simulink model "Aircraft_Simulator_LAT"  (R2019b)
settings: Solver=ode4  StartTime=0.0  StopTime=tfinal  FixedStep=dt  RelTol=1e-3
undefined symbols (not defined in the file or in its folder): aircraft_data, F_gravity_0, initial_conditions, Ixx, Iyy, Izz, m, M0, Matrix_Controls, Matrix_states, s0
libraries: simulink_extras x8, shared6dof x1, aerolibasang x1
settings Model: Creator=yossef  LastModifiedBy=Yousef
settings DataIOCC: ReturnWorkspaceOutputs=off
settings DebuggingCC: ArithmeticOperatorsInVariantConditions=warning
settings SFSimCC: SimUseLocalCustomCode=off  CustomCodeUndefinedFunction=UseInterfaceOnly
settings RTWCC: RTWUseLocalCustomCode=off

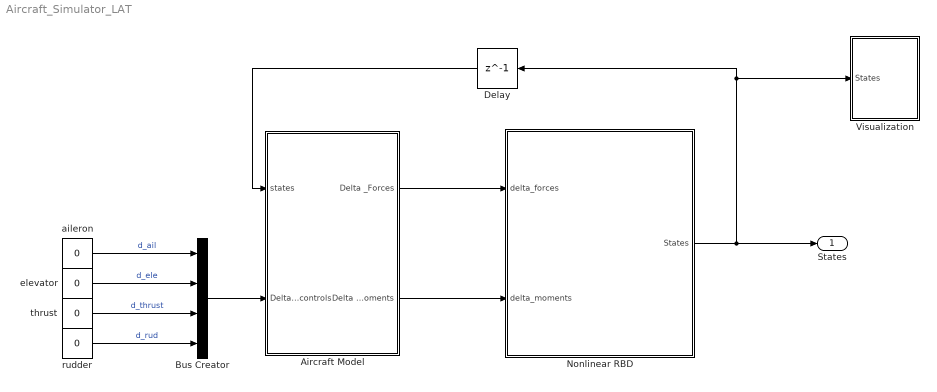
== system Aircraft_Simulator_LAT ==
  Aircraft Model : Subsystem
  Bus Creator : BusCreator  Inputs=4
  Delay : Delay  DelayLength=1  InitialCondition=initial_conditions
  Nonlinear RBD : Subsystem
  Visualization : Subsystem
  aileron : Constant  Value=0
  elevator : Constant  Value=0
  rudder : Constant  Value=0
  thrust : Constant  Value=0
  States : Outport
  wires:
  Delay/1 -> Aircraft Model/1(states)
  Nonlinear RBD/1(States) -> States/1, Delay/1, Visualization/1(States)
  Aircraft Model/1(Delta _Forces) -> Nonlinear RBD/1(delta_forces)
  Aircraft Model/2(Delta _Moments) -> Nonlinear RBD/2(delta_moments)
  aileron/1 -> Bus Creator/1  "d_ail"
  elevator/1 -> Bus Creator/2  "d_ele"
  thrust/1 -> Bus Creator/3  "d_thrust"
  rudder/1 -> Bus Creator/4  "d_rud"
  Bus Creator/1 -> Aircraft Model/2(Delta_controls)

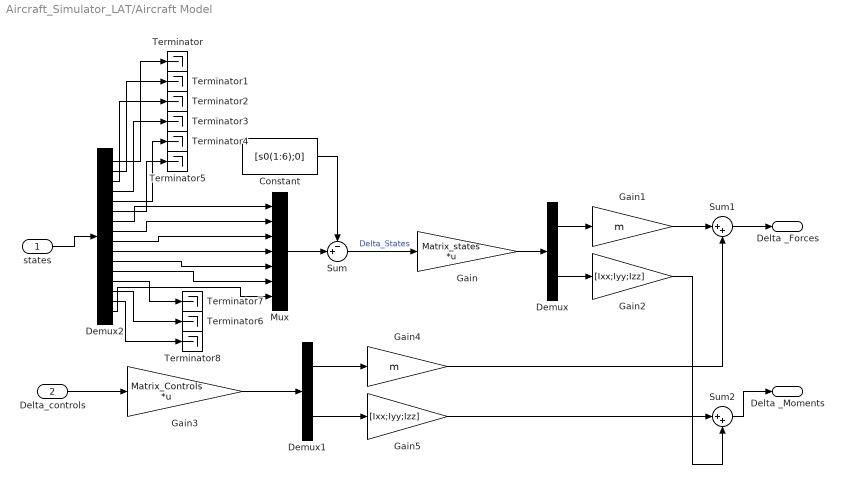
== system Aircraft_Simulator_LAT/Aircraft Model ==
  states : Inport
  Delta_controls : Inport  Port=2
  Constant : Constant  Value=[s0(1:6);0]
  Demux : Demux  Outputs=2
  Demux1 : Demux  Outputs=2
  Demux2 : Demux  Outputs=16
  Gain : Gain  Gain=Matrix_states  Multiplication=Matrix(K*u)
  Gain1 : Gain  Gain=m
  Gain2 : Gain  Gain=[Ixx;Iyy;Izz]
  Gain3 : Gain  Gain=Matrix_Controls  Multiplication=Matrix(K*u)
  Gain4 : Gain  Gain=m
  Gain5 : Gain  Gain=[Ixx;Iyy;Izz]
  Mux : Mux  Inputs=7
  Sum : Sum  Inputs=-+|
  Sum1 : Sum  Inputs=|++
  Sum2 : Sum  Inputs=|++
  Terminator{,1..8} (9 alike) : Terminator
  Delta _Forces : Outport
  Delta _Moments : Outport  Port=2
  wires:
  Mux/1 -> Sum/2
  Constant/1 -> Sum/1
  Sum/1 -> Gain/1  "Delta_States"
  Gain/1 -> Demux/1
  Demux/1 -> Gain1/1
  Demux/2 -> Gain2/1
  Gain2/1 -> Sum2/2
  Gain1/1 -> Sum1/1
  Sum1/1 -> Delta _Forces/1
  Sum2/1 -> Delta _Moments/1
  Delta_controls/1 -> Gain3/1
  Gain3/1 -> Demux1/1
  Demux1/1 -> Gain4/1
  Demux1/2 -> Gain5/1
  Gain4/1 -> Sum1/2
  Gain5/1 -> Sum2/1
  states/1 -> Demux2/1
  Demux2/1 -> Terminator/1
  Demux2/2 -> Terminator1/1
  Demux2/3 -> Terminator2/1
  Demux2/7 -> Mux/1
  Demux2/8 -> Mux/2
  Demux2/9 -> Mux/3
  Demux2/10 -> Mux/4
  Demux2/11 -> Mux/5
  Demux2/12 -> Mux/6
  Demux2/16 -> Mux/7
  Demux2/4 -> Terminator3/1
  Demux2/5 -> Terminator4/1
  Demux2/6 -> Terminator5/1
  Demux2/13 -> Terminator7/1
  Demux2/14 -> Terminator6/1
  Demux2/15 -> Terminator8/1

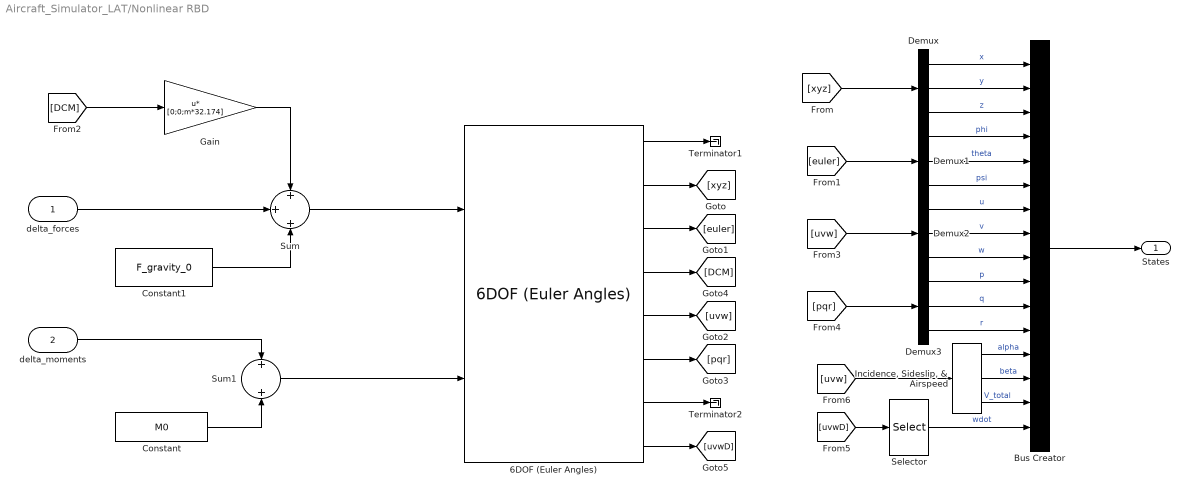
== system Aircraft_Simulator_LAT/Nonlinear RBD ==
  delta_forces : Inport
  delta_moments : Inport  Port=2
  6DOF (Euler Angles) : shared6dof/6DOF (Euler Angles)  units=English (Velocity in ft/s)  mtype=Fixed  rep=Euler Angles  xme_0=aircraft_data(13:15)  Vm_0=aircraft_data(4:6)  eul_0=aircraft_data(10:12)  pm_0=aircraft_data(7:9)  mass_0=m  mass_e=0.5  mass_f=2.0  inertia=I  inertia_e=eye(3)  inertia_f=2*eye(3)  k_quat=1.0  vre_flag=on  abi_flag=off  aMode=0  xme_statename=''  Vm_statename=''  eul_statename=''  quat_statename=''  pm_statename=''  mass_statename=''
      settings: SourceProductBaseCode=AE
  Bus Creator : BusCreator  Inputs=16
  Constant : Constant  Value=M0
  Constant1 : Constant  Value=F_gravity_0
  Demux{,1..3} (4 alike) : Demux  Outputs=3
  Gain : Gain  Gain=[0;0;m*32.174]  Multiplication=Matrix(u*K)
  "Incidence, Sideslip, & Airspeed" : aerolibasang/Incidence, Sideslip, & Airspeed
      settings: SourceProductName=Aerospace Blockset
  Selector : Selector  InputPortWidth=3  IndexOptions=Index vector (dialog)  Indices=[3]  OutputSizes=1
  Sum : Sum  Inputs=+||+||+
  Sum1 : Sum  Inputs=+||+
  Terminator1 : Terminator
  Terminator2 : Terminator
  States : Outport
  wires:
  6DOF (Euler Angles)/4 -> [DCM]
  6DOF (Euler Angles)/1 -> Terminator1/1
  6DOF (Euler Angles)/2 -> [xyz]
  6DOF (Euler Angles)/3 -> [euler]
  6DOF (Euler Angles)/5 -> [uvw]
  6DOF (Euler Angles)/6 -> [pqr]
  6DOF (Euler Angles)/7 -> Terminator2/1
  6DOF (Euler Angles)/8 -> [uvwD]
  Demux/2 -> Bus Creator/2  "y"
  [xyz] -> Demux/1
  Demux/1 -> Bus Creator/1  "x"
  Demux/3 -> Bus Creator/3  "z"
  [uvw] -> Demux2/1
  [pqr] -> Demux3/1
  Demux1/1 -> Bus Creator/4  "phi"
  Demux1/2 -> Bus Creator/5  "theta"
  Demux1/3 -> Bus Creator/6  "psi"
  Demux2/1 -> Bus Creator/7  "u"
  Demux2/2 -> Bus Creator/8  "v"
  Demux2/3 -> Bus Creator/9  "w"
  Demux3/1 -> Bus Creator/10  "p"
  Demux3/2 -> Bus Creator/11  "q"
  Demux3/3 -> Bus Creator/12  "r"
  "Incidence, Sideslip, & Airspeed"/1 -> Bus Creator/13  "alpha"
  "Incidence, Sideslip, & Airspeed"/2 -> Bus Creator/14  "beta"
  "Incidence, Sideslip, & Airspeed"/3 -> Bus Creator/15  "V_total"
  [uvw] -> "Incidence, Sideslip, & Airspeed"/1
  Selector/1 -> Bus Creator/16  "wdot"
  [uvwD] -> Selector/1
  Bus Creator/1 -> States/1
  Constant1/1 -> Sum/3
  [DCM] -> Gain/1
  Gain/1 -> Sum/1
  Sum/1 -> 6DOF (Euler Angles)/1
  delta_forces/1 -> Sum/2
  Constant/1 -> Sum1/2
  delta_moments/1 -> Sum1/1
  Sum1/1 -> 6DOF (Euler Angles)/2
  [euler] -> Demux1/1

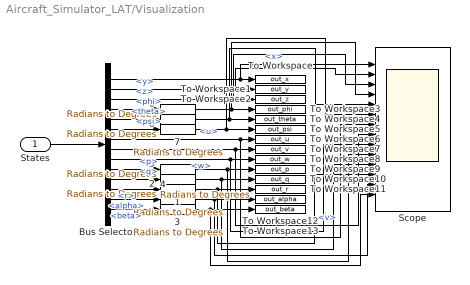
== system Aircraft_Simulator_LAT/Visualization ==
  States : Inport
  {1..8} (8 alike) : simulink_extras/Transformations/Radians to Degrees
  Bus Selector : BusSelector  OutputSignals=x,y,z,phi,theta,psi,u,v,w,p,q,r,alpha,beta
  Scope : Scope  NumInputPorts=14
  To Workspace : ToWorkspace  VariableName=out_x  SampleTime=-1
  To Workspace1 : ToWorkspace  VariableName=out_y  SampleTime=-1
  To Workspace10 : ToWorkspace  VariableName=out_q  SampleTime=-1
  To Workspace11 : ToWorkspace  VariableName=out_r  SampleTime=-1
  To Workspace12 : ToWorkspace  VariableName=out_alpha  SampleTime=-1
  To Workspace13 : ToWorkspace  VariableName=out_beta  SampleTime=-1
  To Workspace2 : ToWorkspace  VariableName=out_z  SampleTime=-1
  To Workspace3 : ToWorkspace  VariableName=out_phi  SampleTime=-1
  To Workspace4 : ToWorkspace  VariableName=out_theta  SampleTime=-1
  To Workspace5 : ToWorkspace  VariableName=out_psi  SampleTime=-1
  To Workspace6 : ToWorkspace  VariableName=out_u  SampleTime=-1
  To Workspace7 : ToWorkspace  VariableName=out_v  SampleTime=-1
  To Workspace8 : ToWorkspace  VariableName=out_w  SampleTime=-1
  To Workspace9 : ToWorkspace  VariableName=out_p  SampleTime=-1
  wires:
  States/1 -> Bus Selector/1
  Bus Selector/1 -> Scope/1, To Workspace/1  "<x>"
  Bus Selector/2 -> Scope/2, To Workspace1/1  "<y>"
  Bus Selector/3 -> Scope/3, To Workspace2/1  "<z>"
  Bus Selector/7 -> Scope/7, To Workspace6/1  "<u>"
  Bus Selector/8 -> Scope/8, To Workspace7/1  "<v>"
  Bus Selector/9 -> Scope/9, To Workspace8/1  "<w>"
  Bus Selector/11 -> 1/1  "<q>"
  1/1 -> Scope/11, To Workspace10/1
  Bus Selector/12 -> 2/1  "<r>"
  Bus Selector/13 -> 3/1  "<alpha>"
  Bus Selector/14 -> 4/1  "<beta>"
  4/1 -> Scope/14, To Workspace13/1
  3/1 -> Scope/13, To Workspace12/1
  2/1 -> Scope/12, To Workspace11/1
  Bus Selector/10 -> 5/1  "<p>"
  5/1 -> Scope/10, To Workspace9/1
  Bus Selector/4 -> 6/1  "<phi>"
  Bus Selector/5 -> 7/1  "<theta>"
  Bus Selector/6 -> 8/1  "<psi>"
  6/1 -> Scope/4, To Workspace3/1
  7/1 -> Scope/5, To Workspace4/1
  8/1 -> Scope/6, To Workspace5/1
